simulink model "Horizontal_Rolling_Tongji_Control"  (R2021b)
settings: Solver=ode15s  StartTime=0.0  StopTime=50  FixedStep=1e-4  MaxStep=1e-4  RelTol=1e-4
values from neighbouring files (symbols this model uses):
  J_1 = m_1*r_1^2/2    (= 0.1)    [Horizontal_Rolling_Tongji.m]
  J_2 = m_2*r_2^2/2    (= 2.5)    [Horizontal_Rolling_Tongji.m]
  mu_d = 0.5    [Horizontal_Rolling_Tongji.m]
  mu_r = mu_s*10^-2    (= 0.0065)    [Horizontal_Rolling_Tongji.m]
  mu_s = 0.65    [Horizontal_Rolling_Tongji.m]
  N = 50    [Horizontal_Rolling_Tongji.m]
  r_1 = 0.2    [Horizontal_Rolling_Tongji.m]
  r_2 = 0.5    [Horizontal_Rolling_Tongji.m]
  resolution = 1e-2    (= 0.01)    [Horizontal_Rolling_Tongji.m]
libraries: cstblocks x4, simulink x1
settings Model: Creator=Gioele  LastModifiedBy=gioele
settings SolverCC: AlgebraicLoopSolver=LineSearch
settings DebuggingCC: SFMachineParentedDataDiag=warning

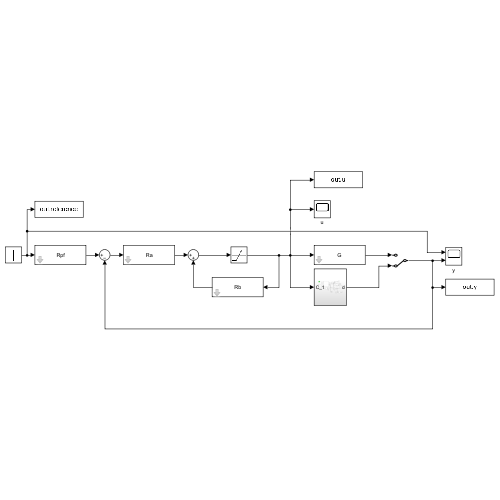
[thumbnail: Simulink's stored preview of the top-level diagram]
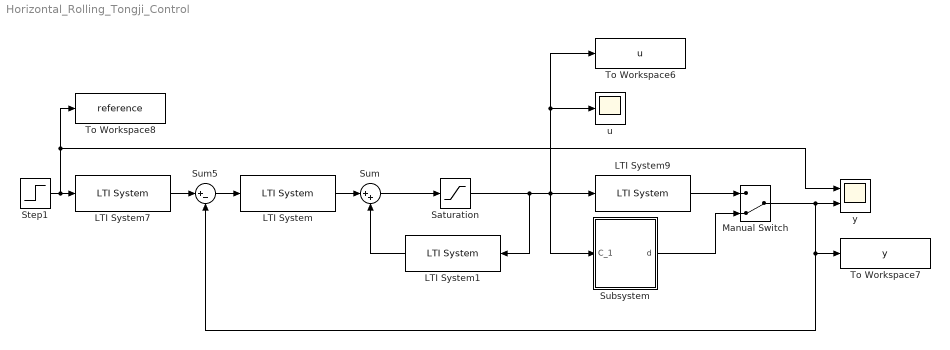
== system Horizontal_Rolling_Tongji_Control ==
  LTI System : cstblocks/LTI System  sys=Ra  IC=[]
  LTI System1 : cstblocks/LTI System  sys=Rb  IC=[]
  LTI System7 : cstblocks/LTI System  sys=Rpf  IC=[]
  LTI System9 : cstblocks/LTI System  sys=G  IC=[]
  Manual Switch : ManualSwitch  CurrentSetting=0
  Saturation : Saturate  UpperLimit=7.7  LowerLimit=-7.7  LinearizeAsGain=off
  Step1 : Step  After=10  SampleTime=0
  Subsystem : Subsystem
  Sum : Sum  Inputs=|++
  Sum5 : Sum  Inputs=|+-
  To Workspace6 : ToWorkspace  VariableName=u  SampleTime=resolution
  To Workspace7 : ToWorkspace  VariableName=y  SampleTime=1e-2
  To Workspace8 : ToWorkspace  VariableName=reference  SampleTime=1e-2
  u : Scope
  y : Scope  NumInputPorts=2
  wires:
  Manual Switch/1 -> To Workspace7/1, Sum5/2, y/2
  Subsystem/1(d) -> Manual Switch/2
  LTI System9/1 -> Manual Switch/1
  Sum/1 -> Saturation/1
  Saturation/1 -> LTI System1/1, To Workspace6/1, u/1, LTI System9/1, Subsystem/1(C_1)
  LTI System/1 -> Sum/1
  LTI System1/1 -> Sum/2
  Sum5/1 -> LTI System/1
  Step1/1 -> LTI System7/1, To Workspace8/1, y/1
  LTI System7/1 -> Sum5/1

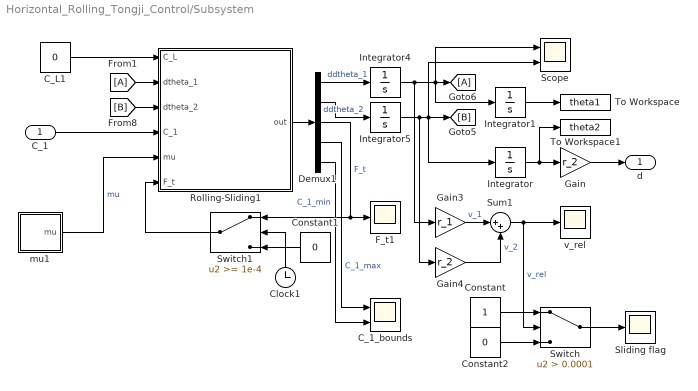
== system Horizontal_Rolling_Tongji_Control/Subsystem ==
  C_1 : Inport
  C_1_bounds : Scope  NumInputPorts=2
  C_L1 : Constant  Value=0
  Clock1 : Clock
  Constant : Constant
  Constant1 : Constant  Value=0
  Constant2 : Constant  Value=0
  Demux1 : Demux  Outputs=5
  F_t1 : Scope
  Gain : Gain  Gain=r_2
  Gain3 : Gain  Gain=r_1
  Gain4 : Gain  Gain=r_2
  Integrator{,1,4..5} (4 alike) : Integrator
  Rolling-Sliding1 : MATLAB Function  TreatAsAtomicUnit=on
  Scope : Scope  NumInputPorts=2
  Sliding flag : Scope
  Sum1 : Sum  Inputs=|++
  Switch : Switch  Criteria=u2 > Threshold  Threshold=0.0001
  Switch1 : Switch  Threshold=1e-4
  To Workspace : ToWorkspace  VariableName=theta1  SampleTime=resolution
  To Workspace1 : ToWorkspace  VariableName=theta2  SampleTime=resolution
  mu1 : Subsystem
  v_rel : Scope
  d : Outport
  wires:
  C_L1/1 -> Rolling-Sliding1/1(C_L)
  Demux1/2 -> Integrator5/1  "ddtheta_2"
  mu1/1(mu) -> Rolling-Sliding1/5(mu)  "mu"
  Demux1/3 -> F_t1/1, Switch1/1  "F_t"
  [A] -> Rolling-Sliding1/2(dtheta_1)
  Clock1/1 -> Switch1/2
  Rolling-Sliding1/1(out) -> Demux1/1
  Switch1/1 -> Rolling-Sliding1/6(F_t)
  Constant1/1 -> Switch1/3
  [B] -> Rolling-Sliding1/3(dtheta_2)
  Demux1/1 -> Integrator4/1  "ddtheta_1"
  C_1/1 -> Rolling-Sliding1/4(C_1)
  Integrator4/1 -> Gain3/1, Integrator1/1, Scope/1, [A]
  Integrator5/1 -> Gain4/1, [B], Scope/2, Integrator/1
  Integrator/1 -> To Workspace1/1, Gain/1
  Gain/1 -> d/1
  Gain4/1 -> Sum1/2  "v_2"
  Gain3/1 -> Sum1/1  "v_1"
  Sum1/1 -> Switch/2, v_rel/1  "v_rel"
  Constant/1 -> Switch/1
  Constant2/1 -> Switch/3
  Switch/1 -> Sliding flag/1
  Demux1/4 -> C_1_bounds/1  "C_1_max"
  Demux1/5 -> C_1_bounds/2  "C_1_min"
  Integrator1/1 -> To Workspace/1

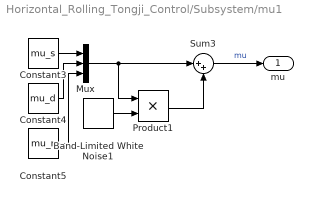
== system Horizontal_Rolling_Tongji_Control/Subsystem/mu1 ==
  Band-Limited White Noise1 : simulink/Sources/Band-Limited White Noise  Cov=[0.000001]  Ts=0.1  seed=[23341]
  Constant3 : Constant  Value=mu_s
  Constant4 : Constant  Value=mu_d
  Constant5 : Constant  Value=mu_r
  Mux : Mux  Inputs=3
  Product1 : Product
  Sum3 : Sum  Inputs=|++
  mu : Outport
  wires:
  Sum3/1 -> mu/1  "mu"
  Constant5/1 -> Mux/3
  Constant4/1 -> Mux/2
  Product1/1 -> Sum3/2
  Constant3/1 -> Mux/1
  Mux/1 -> Sum3/1, Product1/1
  Band-Limited White Noise1/1 -> Product1/2

== matlab function Horizontal_Rolling_Tongji_Control/Subsystem/Rolling-Sliding1 ==
  data: C_L input; dtheta_1 input; dtheta_2 input; C_1 input; r_1 parameter; r_2 parameter; J_1 parameter; J_2 parameter; N parameter; mu input; F_t input; out output
function out = fcn(C_L,dtheta_1,dtheta_2,C_1,r_1,r_2,J_1,J_2,N,mu,F_t)
% function out = fcn(dtheta_1,dtheta_2,ddtheta_1,ddtheta_2,tau,r_1,r_2,J_1,J_2,N, mu)

mu_s_n = mu(1);
mu_d_n = mu(2);
mu_r_n = mu(3);

if abs(dtheta_1) > 0.1
    C_rf1 = - sign(dtheta_1)*mu_r_n*N;
else
%     if abs(C_1) < mu_r_n*P_n
%         C_rf1 = - C_1;
%     else
%         C_rf1 = - sign(dtheta_1)*mu_r_n*P_n;
%     end
    C_rf1 = 0;
end

if abs(dtheta_2) > 0.1
    C_rf2 = - sign(dtheta_2)*mu_r_n*N;
else
%     if abs(- F_t*r_2) < mu_r_n*P_n
%         C_rf2 = - (- F_t*r_2);
%     else
%         C_rf2 = - sign(dtheta_2)*mu_r_n*P_n;
%     end
    C_rf2 = 0;
end

% if abs(dtheta_1) > 0.001
%     C_rf1 = - sign(dtheta_1)*mu_r_n*N;
% else
%     if abs(C_1) < mu_r_n*N
%         C_rf1 = - C_1;
%     else
%         C_rf1 = - sign(dtheta_1)*mu_r_n*N;
%     end
% end
% C_rf1 = - sign(dtheta_1)*mu_r_n*N;
% if abs(dtheta_2) > 0.001
%     C_rf2 = - sign(dtheta_2)*mu_r_n*N;
% else
%     if abs(- F_t*r_2) < mu_r_n*N
%         C_rf2 = - (- F_t*r_2);
%     else
%         C_rf2 = - sign(dtheta_2)*mu_r_n*N;
%     end
% end
% C_rf2 = - sign(dtheta_2)*mu_r_n*N;

if (-0.001 < dtheta_1*r_1 + dtheta_2*r_2) && (dtheta_1*r_1 + dtheta_2*r_2 < 0.001)
    % Condition should be (dtheta_1*r_1 + dtheta_2*r_2 == 0) but need
    % tolerance for simulation reasons
    F_t = (C_1*J_2*r_1 + C_rf1*J_2*r_1 + C_rf2*J_1*r_2 + C_L*J_1*r_2)/(J_2*r_1^2 + J_1*r_2^2);
    % Pure rolling case
    if (abs(F_t) > mu_s_n*N)
        F_t = sign(dtheta_1*r_1 + dtheta_2*r_2)*mu_d_n*N;
        % Transition from Rolling to Rolling with sliding
    end
else
    F_t = sign(dtheta_1*r_1 + dtheta_2*r_2)*mu_d_n*N;
    % Rolling with sliding case
end

ddtheta_1 = (C_1 + C_rf1 - F_t*r_1)/(J_1);
ddtheta_2 = (- F_t*r_2 + C_rf2 + C_L)/(J_2);

C_1_max = (mu_s_n*N*(J_2*r_1^2+J_1*r_2^2)-(C_rf2+C_L)*J_1*r_2)/(J_2*r_1)-C_rf1;
C_1_min = (-mu_s_n*N*(J_2*r_1^2+J_1*r_2^2)-(C_rf2+C_L)*J_1*r_2)/(J_2*r_1)-C_rf1;


out = [ddtheta_1,ddtheta_2,F_t,C_1_max,C_1_min];
